simulink model "MRAC_P1_Projection"  (R2019b)
settings: Solver=ode45  StartTime=0.0  StopTime=1500  RelTol=1e-5
undefined symbols (not defined in the file or in its folder): sigbuilder_block
libraries: slctrlblks x3, simulink x2
settings Model: Creator=Henry  LastModifiedBy=Kevin
settings SFSimCC: CustomCodeUndefinedFunction=UseInterfaceOnly

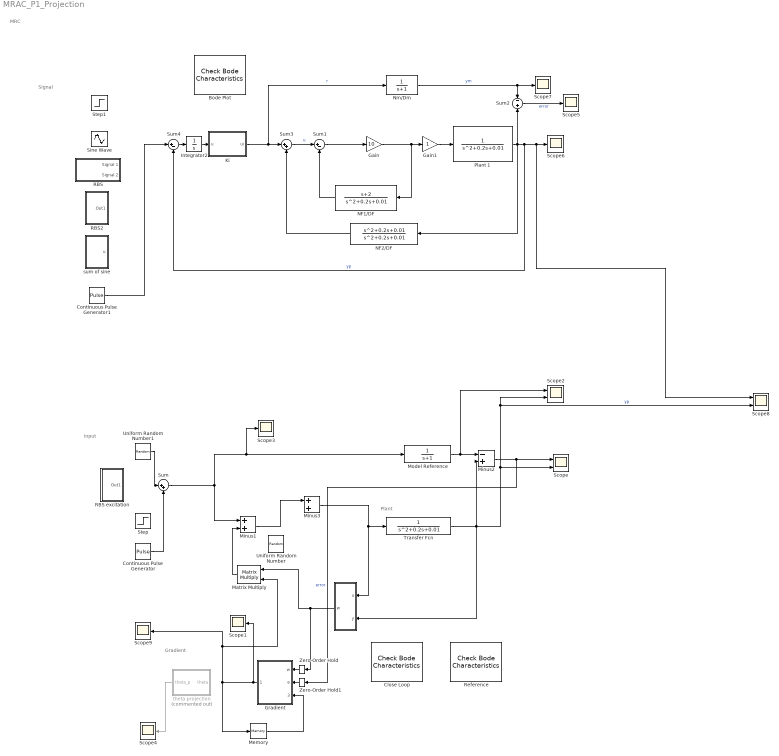
== system MRAC_P1_Projection ==
  note: MRC
  note: Input
  note: Plant
  note: Gradient
  note: Signal
  " " : Subsystem
  Bode Plot : slctrlblks/Model Verification/Check Bode  Characteristics  InstantiateOnLoad=on  SaveOperatingPoints=off  LinearizationIOs={'/Gain1', 1, 'in', 'off', '';'/Plant 1', 1, 'out', 'on', ''}  LinearizeAt=SnapshotTimes  SnapshotTimes=[0]  TriggerType=rising  SampleTime=auto  RateConversionMethod=zoh  PreWarpFreq=10  UseExactDelayModel=off  UseFullBlockNameLabels=off  UseBusSignalLabels=off  enabled=on  stopWhenAssertionFail=off  export=off  ViewDlgPos=[1981 -205.666666666667 1445.33333333333 714]  OpenViewOnLoad=off  LaunchViewOnOpen=off  FrequencyUnits=rad/s  MagnitudeUnits=dB  PhaseUnits=deg  TimeUnits=seconds  EnableUpperBound=off  UpperBoundFrequencies=[]  UpperBoundMagnitudes=[]  EnableLowerBound=off  LowerBoundFrequencies=[]  LowerBoundMagnitudes=[]
      settings: SourceProductName=Simulink Control Design
  Close Loop : slctrlblks/Model Verification/Check Bode  Characteristics  InstantiateOnLoad=on  SaveOperatingPoints=off  LinearizationIOs={'/Transfer Fcn', 1, 'out', 'off', '';'/Minus1', 1, 'in', 'off', ''}  LinearizeAt=SnapshotTimes  SnapshotTimes=[0]  TriggerType=rising  SampleTime=auto  RateConversionMethod=zoh  PreWarpFreq=10  UseExactDelayModel=off  UseFullBlockNameLabels=off  UseBusSignalLabels=off  enabled=on  stopWhenAssertionFail=off  export=off  ViewDlgPos=[100 200 510 390]  OpenViewOnLoad=off  LaunchViewOnOpen=on  FrequencyUnits=rad/s  MagnitudeUnits=dB  PhaseUnits=deg  TimeUnits=seconds  EnableUpperBound=off  UpperBoundFrequencies=[]  UpperBoundMagnitudes=[]  EnableLowerBound=off  LowerBoundFrequencies=[]  LowerBoundMagnitudes=[]
      settings: SourceProductName=Simulink Control Design
  Continuous Pulse Generator : DiscretePulseGenerator  PulseType=Time based  Period=60  PulseWidth=50
  Continuous Pulse Generator1 : DiscretePulseGenerator  PulseType=Time based  Period=1  PulseWidth=50
  Gain : Gain  Gain=10
  Gain1 : Gain
  Gradient : MATLAB Function  TreatAsAtomicUnit=on
  Integrator2 : Integrator
  Ki : MATLAB Function  TreatAsAtomicUnit=on
  Matrix Multiply : Product  Multiplication=Matrix(*)
  Memory : Memory  InitialCondition=[0 0 0 0 0]'  InheritSampleTime=on
  Minus1 : Sum
  Minus2 : Sum  Inputs=-+
  Minus3 : Sum
  Model Reference : TransferFcn  Denominator=[1 1]
  NF1/DF : TransferFcn  Numerator=[1 2]  Denominator=[1 0.2 0.01]
  NF2/DF : TransferFcn  Numerator=[1 0.2 0.01]  Denominator=[1 0.2 0.01]
  "Nm/Dm " : TransferFcn  Denominator=[1 1]
  Plant 1 : TransferFcn  Denominator=[1 ,0.2 ,0.01]
  "RBS " : Subsystem  Tag=STV Subsys  LoadFcn=sigbuilder_block('load');  StartFcn=sigbuilder_block('start');  StopFcn=sigbuilder_block('stop');  ClipboardFcn=sigbuilder_block('clipboard');  mask(Sigbuilder block){tuvar=[0:10]}
      mask help: Simulink:masks:SigbuilderBlock_MD
      mask init:
      | if ~strcmp(get_param(bdroot(gcbh),'SimulationStatus'),'stopped') tuvar = sigbuilder_block('maskInit'); end
      settings: CopyFcn=sigbuilder_block('copy');  DeleteFcn=sigbuilder_block('delete');  ModelCloseFcn=sigbuilder_block('modelClose');  PreSaveFcn=sigbuilder_block('preSave');  PauseFcn=sigbuilder_block('pause');  ContinueFcn=sigbuilder_block('continue');  NameChangeFcn=sigbuilder_block('namechange');  OpenFcn=sigbuilder_block('open',[215 62.5 550.5 362.5 ]);  CloseFcn=sigbuilder_block('close');
      mask Display: plot(0, 0, 100, 100,[2, 2, 32, 32, 2], [68, 8, 8, 68, 68],[32, 2], [38, 38], [32, 19, 2],[53, 60, 44], [32, 17, 17, 2],[16, 16, 31, 31]);txt = getActiveGroup(gcbh);text(2, 100, txt,'verticalAlignment', 'top');
  RBS excitation : Subsystem
  RBS2 : Subsystem
  Reference : slctrlblks/Model Verification/Check Bode  Characteristics  InstantiateOnLoad=on  SaveOperatingPoints=off  LinearizationIOs={'/Model Reference', 1, 'out', 'off', '';'/Step', 1, 'in', 'off', ''}  LinearizeAt=SnapshotTimes  SnapshotTimes=[0]  TriggerType=rising  SampleTime=auto  RateConversionMethod=zoh  PreWarpFreq=10  UseExactDelayModel=off  UseFullBlockNameLabels=off  UseBusSignalLabels=off  enabled=on  stopWhenAssertionFail=off  export=off  ViewDlgPos=[100 200 510 390]  OpenViewOnLoad=off  LaunchViewOnOpen=on  FrequencyUnits=rad/s  MagnitudeUnits=dB  PhaseUnits=deg  TimeUnits=seconds  EnableUpperBound=off  UpperBoundFrequencies=[]  UpperBoundMagnitudes=[]  EnableLowerBound=off  LowerBoundFrequencies=[]  LowerBoundMagnitudes=[]
      settings: SourceProductName=Simulink Control Design
  Scope : Scope  NumInputPorts=2
  Scope{1,3..7,9} (7 alike) : Scope
  Scope2 : Scope  NumInputPorts=2
  Scope8 : Scope  NumInputPorts=2
  Sine Wave : Sin  Frequency=0.1  SampleTime=0
  Step : Step  SampleTime=0
  Step1 : Step  SampleTime=0
  Sum : Sum  Inputs=|++
  Sum1 : Sum  Inputs=|+-
  Sum2 : Sum  Inputs=-+
  Sum3 : Sum  Inputs=|++
  Sum4 : Sum  Inputs=|+-
  Transfer Fcn : TransferFcn  Denominator=[1 ,0.2 ,0.01]
  Uniform Random Number : UniformRandomNumber  Minimum=-0.1  Maximum=0.1  SampleTime=0.1
  Uniform Random Number1 : UniformRandomNumber  Minimum=-0.1  Maximum=0.1  SampleTime=0.1
  Zero-Order Hold : ZeroOrderHold  SampleTime=0.01
  Zero-Order Hold1 : ZeroOrderHold  SampleTime=0.01
  sum of sine : Subsystem
  theta projection : MATLAB Function  Commented=on  TreatAsAtomicUnit=on
  wires:
  Model Reference/1 -> Scope2/1, Minus2/1
  Transfer Fcn/1 -> " "/2("y "), Scope8/2, Scope2/2, Scope/2, Minus2/2  "yp"
  Sum/1 -> Minus1/1, Scope3/1, Model Reference/1
  Minus3/1 -> " "/1("u "), Transfer Fcn/1
  Matrix Multiply/1 -> Minus1/2
  " "/1(w) -> Zero-Order Hold/1, Matrix Multiply/1
  Minus2/1 -> Zero-Order Hold1/1, Scope/1  "error"
  Memory/1 -> Gradient/3(theta_k)
  Minus1/1 -> Minus3/1
  Continuous Pulse Generator/1 -> Sum/2
  NF2/DF/1 -> Sum3/2
  NF1/DF/1 -> Sum1/2
  Gain1/1 -> Plant 1/1
  Gain/1 -> Gain1/1, NF1/DF/1
  Continuous Pulse Generator1/1 -> Sum4/1
  Sum1/1 -> Gain/1
  Sum4/1 -> Integrator2/1
  Integrator2/1 -> Ki/1(u)
  Sum2/1 -> Scope5/1  "error"
  Plant 1/1 -> Scope8/1, Scope6/1, Sum4/2, NF2/DF/1, Sum2/2  "yp"
  Ki/1(ui) -> "Nm/Dm "/1, Sum3/1  "r"
  "Nm/Dm "/1 -> Scope7/1, Sum2/1  "ym"
  Sum3/1 -> Sum1/1  "u"
  Gradient/1(theta_k1) -> Memory/1, Scope9/1, Matrix Multiply/2, Scope1/1
  theta projection/1(theta_p) -> Scope4/1
  Zero-Order Hold/1 -> Gradient/1(w)
  Zero-Order Hold1/1 -> Gradient/2(e)
  Uniform Random Number1/1 -> Sum/1

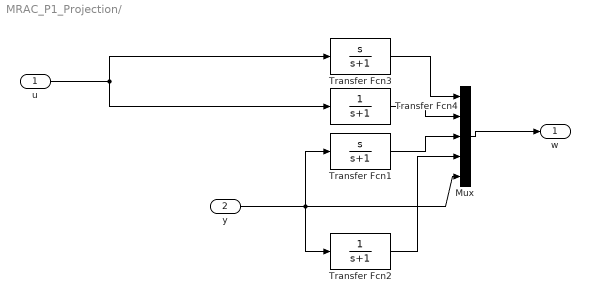
== system MRAC_P1_Projection/  ==
  "u " : Inport
  "y " : Inport  Port=2
  Mux : Mux  Inputs=5
  Transfer Fcn1 : TransferFcn  Numerator=[1 0]  Denominator=[1 1]
  Transfer Fcn2 : TransferFcn  Denominator=[1 1]
  Transfer Fcn3 : TransferFcn  Numerator=[1 0]  Denominator=[1 1]
  Transfer Fcn4 : TransferFcn  Denominator=[1 1]
  w : Outport
  wires:
  Transfer Fcn1/1 -> Mux/3
  "u "/1 -> Transfer Fcn3/1, Transfer Fcn4/1
  Mux/1 -> w/1
  "y "/1 -> Mux/5, Transfer Fcn2/1, Transfer Fcn1/1
  Transfer Fcn2/1 -> Mux/4
  Transfer Fcn3/1 -> Mux/1
  Transfer Fcn4/1 -> Mux/2

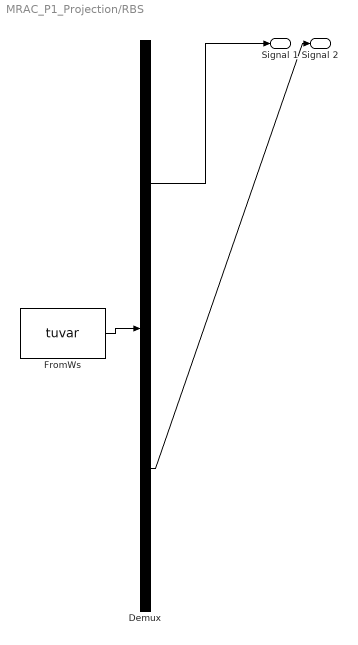
== system MRAC_P1_Projection/RBS  ==
  Demux : Demux  Tag=STV Demux  Outputs=2
  FromWs : FromWorkspace  Tag=STV FromWs  VariableName=tuvar  SampleTime=0
      SigBuilderData=|
      | common.afterFinalStr = 'Extrapolate'
      | common.sampleTime = 0
      | dataSet.timeRange = [0 10]
      | dataSet.name = 'Group 1'
      | sbobj.Groups.Name = 'Group 1'
      | sbobj.Groups.Signals(1).Name = 'Signal 1'
      | sbobj.Groups.Signals(1).XData = [0 4 4 6 6 10]
      | sbobj.Groups.Signals(1).YData = [0 0 1 1 0 0]
      | sbobj.Groups.Signals(2).Name = 'Signal 2'
      | sbobj.Groups.Signals(2).XData = [0 0.2 0.2 0.3 0.3 0.5 0.5 0.7 0.7 1 1 1.1 1.1 1.3 1.3 1.4 1.4 1.5 1.5 1.7 1.7 2.1 2.1 2.2 2.2 2.7 2.7 2.8 2.8 2.9 2.9 3 3 3.1 3.1 3.5 3.5 3.7 3.7 3.8 3.8 3.9 3.9 4.2 4.2 4.4 4.4 4.7 4.7 5 5 5.1 5.1 5.3 5.3 5.6 5.6 5.7 5.7 5.8 5.8 5.9 5.9 6 6 6.1 6.1 6.2 6.2 6.7 6.7 7 7 7.1 7.1 7.2 7.2 7.3 7.3 7.4 7.4 7.5 7.5 7.8 7.8 7.9 7.9 8.1 8.1 8.5 8.5 8.6 8.6 8.8 8.8 8.9 8.9 9 9 9.2 9.2 9.5 9.5 9.6 9.6 9.7 9.7 10]
      | sbobj.Groups.Signals(2).YData = [1 1 0 0 1 1 0 0 1 1 0 0 1 1 0 0 1 1 0 0 1 1 0 0 1 1 0 0 1 1 0 0 1 1 0 0 1 1 0 0 1 1 0 0 1 1 0 0 1 1 0 0 1 1 0 0 1 1 0 0 1 1 0 0 1 1 0 0 1 1 0 0 1 1 0 0 1 1 0 0 1 1 0 0 1 1 0 0 1 1 0 0 1 1 0 0 1 1 0 0 1 1 0 0 1 1 0 0]
  Signal 1 : Outport  Tag=STV Outport
  Signal 2 : Outport  Tag=STV Outport  Port=2
  wires:
  Demux/1 -> Signal 1/1
  FromWs/1 -> Demux/1
  Demux/2 -> Signal 2/1

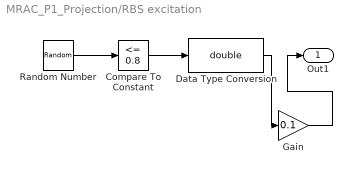
== system MRAC_P1_Projection/RBS excitation ==
  Compare To Constant : simulink/Logic and Bit Operations/Compare To Constant  relop=<=  const=0.8  OutDataTypeStr=boolean
  Data Type Conversion : DataTypeConversion  OutDataTypeStr=double
  Gain : Gain  Gain=0.1
  Random Number : RandomNumber  Mean=1  SampleTime=10
  Out1 : Outport
  wires:
  Random Number/1 -> Compare To Constant/1
  Compare To Constant/1 -> Data Type Conversion/1
  Data Type Conversion/1 -> Gain/1
  Gain/1 -> Out1/1

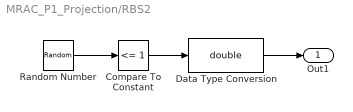
== system MRAC_P1_Projection/RBS2 ==
  Compare To Constant : simulink/Logic and Bit Operations/Compare To Constant  relop=<=  const=1  OutDataTypeStr=boolean
  Data Type Conversion : DataTypeConversion  OutDataTypeStr=double
  Random Number : RandomNumber  Mean=1  SampleTime=10
  Out1 : Outport
  wires:
  Random Number/1 -> Compare To Constant/1
  Compare To Constant/1 -> Data Type Conversion/1
  Data Type Conversion/1 -> Out1/1

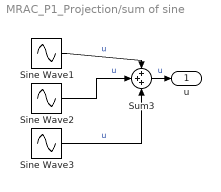
== system MRAC_P1_Projection/sum of sine ==
  Sine Wave1 : Sin  Frequency=0.1  Phase=0.1  SampleTime=0
  Sine Wave2 : Sin  SampleTime=0
  Sine Wave3 : Sin  Frequency=2  SampleTime=0
  Sum3 : Sum  Inputs=+++
  u : Outport
  wires:
  Sine Wave3/1 -> Sum3/3  "u"
  Sine Wave1/1 -> Sum3/1  "u"
  Sum3/1 -> u/1  "u"
  Sine Wave2/1 -> Sum3/2  "u"

== matlab function MRAC_P1_Projection/theta projection ==
  data: theta input; theta_p output
function theta_p = fcn(theta)
theta_max = [0.017 0.078 0 -0.01 -1]'+[0.1 0.7 0.1 0.1 1]';
theta_min = [0.017 0.078 0 -0.01 -1]'-[0.017 0.078 0.1 0.1 0.1]';

max_proj = [0.017 0.078 0 -0.01 -1]';
min_proj = [0.017 0.078 0 -0.01 -1]';

if theta < theta_max
    if theta > theta_min
       theta_p = theta;
    else
        theta_p = min_proj;
    end
else
    theta_p = max_proj;
end

== matlab function MRAC_P1_Projection/Gradient ==
  data: w input; theta_k1 output; e input; theta_k input
function theta_k1 = fcn(w, e, theta_k)
%alpha = 0.1;
%I = eye(5);
% gamma = alpha*I;
gamma = 0.0001;
m = 1; %norms

%projection modification
% theta_max = 1.5*[1 1 1 1 1]';
% theta_min = -1.4*[1 1 1 1 1]';
%theta_star = [0.017 0.078 0 -0.01 -1]';
%theta_max = [0.017 0.078 0 -0.01 -1]'+[0.5 0.7 0.1 0.1 3]';
%theta_min = [0.017 0.078 0 -0.01 -1]'-[0.117 0.178 0.5 0.3 0.8]';
theta_max = [0.517  0.778  0.1  0.09  2]';
theta_min = [-0.1 -0.1  -0.5 -0.31  -1.8]';
%theta_dot = -gamma*w*e;
% if theta < theta_max
%     if theta > theta_min
%         theta_dot = -gamma*w*e;
%     else
%         theta_dot = [0 0 0 0 0]';
%         %theta_dot = gamma*w*e;
%     end
% else
%     theta_dot = [0 0 0 0 0]';
%     %theta_dot = gamma*w*e;

%discrete version
theta_k1 = theta_k -gamma*e*w;
for i = 1:5
    if theta_k1(i) < theta_max(i)
        if theta_k1(i) > theta_min(i)
            continue;
        else
        theta_k1(i) = theta_min(i);
        end
    else
        theta_k1(i) = theta_max(i);
    end
end
end

== matlab function MRAC_P1_Projection/Ki ==
  data: u input; ui output
function ui = fcn(u)
 coder.extrinsic("ss","place","matsplit",'ctrb');
% [b2, b1, b0, a1, a0] = matsplit(theta);
ui = 0;
A = [0 1; -0.01 -0.2];
B = [0 1]';
C = [1 0];

o = [0 0]';
A1 = [A o;C 0];
B1 = [B;0];
p = [-.1+0.69805i -.1-0.69805i -1];
K1 = place(A1,B1,p);
Ki = [K1(3)];
ui = Ki*u;
